simulink model "hdl_fft_sim"  (R2019a)
settings: Solver=VariableStepAuto  StartTime=0.0  StopTime=1024  RelTol=1e-3
undefined symbols (not defined in the file or in its folder): FFT, Wideband_FFT_slim
libraries: xbsIndex_r4 x22, casper_library_misc x1
settings Model: Creator=kocz  LastModifiedBy=kocz

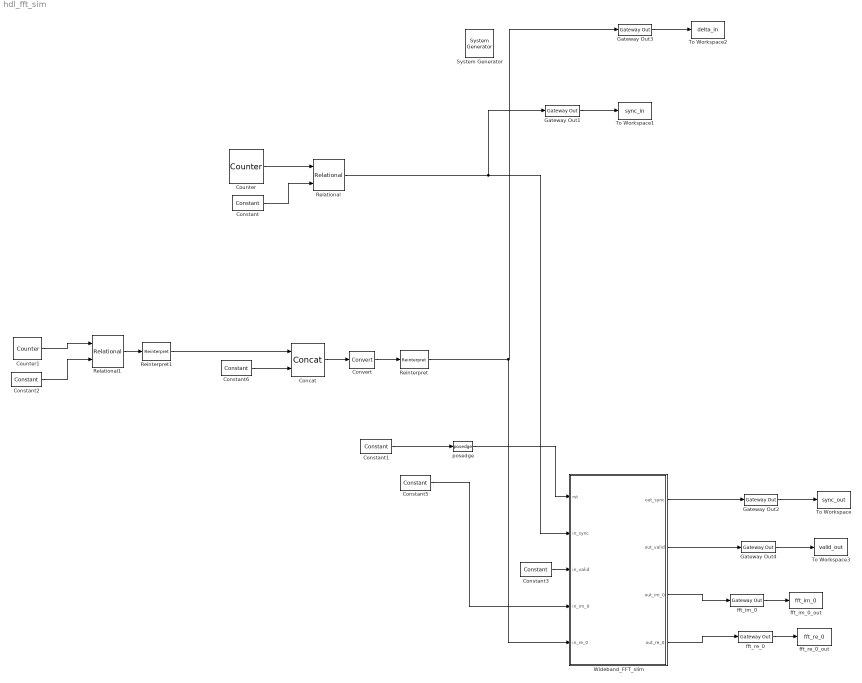
== system hdl_fft_sim ==
  " System Generator" : xbsIndex_r4/ System Generator  Tag=genX  xilinxfamily=kintex7  part=xc7k325t  speed=-3  package=fbg676  synthesis_tool=Vivado  clock_wrapper=Clock Enables  directory=./netlist  proj_type=Vivado  Synth_file=Vivado Synthesis Defaults  Impl_file=Vivado Implementation Defaults  testbench=off  simulink_period=1  sysclk_period=10  dcm_input_clock_period=10  incr_netlist=off  trim_vbits=Everywhere in SubSystem  dbl_ovrd=According to Block Masks  core_generation=According to Block Masks  run_coregen=off  deprecated_control=off  eval_field=0  block_type=sysgen
  Concat : xbsIndex_r4/Concat  num_inputs=2  dbl_ovrd=off  block_type=concat
  Constant : xbsIndex_r4/Constant  const=1  gui_display_data_type=Fixed-point  arith_type=Unsigned  n_bits=32  bin_pt=0  preci_type=Single  exp_width=8  frac_width=24  explicit_period=on  period=1  equ=P=C  opselect=C  inp2=PCIN>>17  opr=+  inp1=P  carry=CIN  dbl_ovrd=off  block_type=constant
  Constant1 : xbsIndex_r4/Constant  const=1  gui_display_data_type=Boolean  arith_type=Boolean  n_bits=16  bin_pt=14  preci_type=Single  exp_width=8  frac_width=24  explicit_period=on  period=1  equ=P=C  opselect=C  inp2=PCIN>>17  opr=+  inp1=P  carry=CIN  dbl_ovrd=off  block_type=constant
  Constant2 : xbsIndex_r4/Constant  const=1  gui_display_data_type=Fixed-point  arith_type=Unsigned  n_bits=32  bin_pt=0  preci_type=Single  exp_width=8  frac_width=24  explicit_period=on  period=1  equ=P=C  opselect=C  inp2=PCIN>>17  opr=+  inp1=P  carry=CIN  dbl_ovrd=off  block_type=constant
  Constant3 : xbsIndex_r4/Constant  const=1  gui_display_data_type=Boolean  arith_type=Boolean  n_bits=16  bin_pt=14  preci_type=Single  exp_width=8  frac_width=24  explicit_period=on  period=1  equ=P=C  opselect=C  inp2=PCIN>>17  opr=+  inp1=P  carry=CIN  dbl_ovrd=off  block_type=constant
  Constant5 : xbsIndex_r4/Constant  const=0  gui_display_data_type=Fixed-point  arith_type=Signed (2's comp)  n_bits=18  bin_pt=17  preci_type=Single  exp_width=8  frac_width=24  explicit_period=on  period=1  equ=P=C  opselect=C  inp2=PCIN>>17  opr=+  inp1=P  carry=CIN  dbl_ovrd=off  block_type=constant
  Constant6 : xbsIndex_r4/Constant  const=0  gui_display_data_type=Fixed-point  arith_type=Unsigned  n_bits=4  bin_pt=0  preci_type=Single  exp_width=8  frac_width=24  explicit_period=on  period=1  equ=P=C  opselect=C  inp2=PCIN>>17  opr=+  inp1=P  carry=CIN  dbl_ovrd=off  block_type=constant
  Convert : xbsIndex_r4/Convert  gui_display_data_type=Fixed-point  arith_type=Unsigned  n_bits=18  bin_pt=0  float_type=Single  exp_bits=8  fraction_bits=24  quantization=Truncate  overflow=Wrap  en=off  latency=2  pipeline=off  dbl_ovrd=off  block_type=convert
  Counter : xbsIndex_r4/Counter  cnt_type=Free Running  cnt_to=Inf  operation=Up  start_count=0  cnt_by_val=1  arith_type=Unsigned  n_bits=64  bin_pt=0  load_pin=off  rst=off  en=off  explicit_period=on  period=1  use_behavioral_HDL=off  implementation=Fabric  dbl_ovrd=off  block_type=counter
  Counter1 : xbsIndex_r4/Counter  cnt_type=Free Running  cnt_to=Inf  operation=Up  start_count=0  cnt_by_val=1  arith_type=Unsigned  n_bits=6  bin_pt=0  load_pin=off  rst=off  en=off  explicit_period=on  period=1  use_behavioral_HDL=off  implementation=Fabric  dbl_ovrd=off  block_type=counter
  Gateway Out{1..4} (4 alike) : xbsIndex_r4/Gateway Out  inherit_from_input=off  hdl_port=on  rows=1  columns=1  UseAsDAC=off  DACChannel='1'  interface=None  automatic_assignment=on  address_offset=hex2dec('00')  intf_name=''  intf_description=''  timing_constraint=None  locs_specified=off  LOCs={}  io_standard={}  block_type=gatewayout
  Reinterpret : xbsIndex_r4/Reinterpret  force_arith_type=on  arith_type="Signed  (2's comp)"  force_bin_pt=on  bin_pt=17  block_type=reinterpret
  Reinterpret1 : xbsIndex_r4/Reinterpret  force_arith_type=on  arith_type=Unsigned  force_bin_pt=on  bin_pt=0  block_type=reinterpret
  Relational : xbsIndex_r4/Relational  mode=a=b  op_type=Bool  en=off  latency=1  dbl_ovrd=off  block_type=relational
  Relational1 : xbsIndex_r4/Relational  mode=a=b  op_type=Bool  en=off  latency=0  dbl_ovrd=off  block_type=relational
  To Workspace : ToWorkspace  VariableName=sync_out  SampleTime=-1
      settings: Save2DSignal=2-D array (concatenate along first dimension)
  To Workspace1 : ToWorkspace  VariableName=sync_in  SampleTime=-1
      settings: Save2DSignal=2-D array (concatenate along first dimension)
  To Workspace2 : ToWorkspace  VariableName=delta_in  SampleTime=-1
      settings: Save2DSignal=2-D array (concatenate along first dimension)
  To Workspace3 : ToWorkspace  VariableName=valid_out  SampleTime=-1
      settings: Save2DSignal=2-D array (concatenate along first dimension)
  Wideband_FFT_slim : Subsystem  AncestorBlock=FFT/Wideband_FFT_slim  mask{use_separate=on, use_fft_shift=off, use_reorder=on, nof_chan=0, wb_factor=1, twiddle_offset=0, nof_points=1024, in_dat_w=8, out_dat_w=13, out_gain_w=0, stage_dat_w=16, guard_enable=off, guard_w=2, xtra_dat_sigs=off}
      mask prompts: use_separate "Separate complex in/out ports?"; use_fft_shift "Apply FFT shifting"; use_reorder "Reorder output"; nof_chan "Nof channels (time mux inputs)"; wb_factor "Wideband factor"; twiddle_offset "Twiddle offsets"; nof_points "Number of points"; in_dat_w "Input data width"; out_dat_w "Ouput data width"; out_gain_w "Output gain width"; stage_dat_w "Stage data width"; guard_enable "Guard enable"; guard_w "Guard bit width"; xtra_dat_sigs "Use extended data signals?"
      mask init:
      | Simulink.Block.eval([gcb, '/wb_fft_slim']);
      | 
      | wb_slim_subsys2bb_knit();
      | 
      | if strcmp(guard_enable,'on')
      |     guard_w = 2;
      | end
      mask Callback use_separate:
      | % Control parameter visiblity
      | 
      | % Get the value of the Enable Bias checkbox
      | % unchecked = 'off'
      | % checked = 'on'
      | enab = get_param(gcb,'use_separate');
      | 
      | % Set the 'MaskVisibilities' property for each parameters
      | if strcmp(enab,'on')
      |     set_param(gcb,'MaskEnables',{'on','off','off','on','on','on','on','on','on','on','on','on','on','on'});
      |     set_param(gcb,'use_reorder','on');
      |     set_param(gcb,'use_fft_shift','off');
      | else
      |     set_param(gcb,'MaskEnables',{'on','on','on','on','on','on','on','on','on','on','on','on','off','on'});
      | end
      | 
      | % Note that the value of the bias is not handled here.
      | % See the Initialization tab
      mask Callback use_fft_shift:
      | % Control parameter visiblity
      | 
      | % Get the value of the Enable Bias checkbox
      | % unchecked = 'off'
      | % checked = 'on'
      | enab = get_param(gcb,'use_fft_shift');
      | 
      | % Set the 'MaskVisibilities' property for each parameters
      | if strcmp(enab,'on')
      |     set_param(gcb,'MaskEnables',{'on','on','off','on','on','on','on','on','on','on','on','on','off','on'});
      |     set_param(gcb,'use_reorder','on');
      | else
      |     set_param(gcb,'MaskEnables',{'on','on','on','on','on','on','on','on','on','on','on','on','off','on'});
      | end
      | 
      | % Note that the value of the bias is not handled here.
      | % See the Initialization tab
      mask Callback guard_enable:
      | % Control parameter visiblity
      | 
      | % Get the value of the Enable Bias checkbox
      | % unchecked = 'off'
      | % checked = 'on'
      | enab = get_param(gcb,'guard_enable');
      | 
      | % Set the 'MaskVisibilities' property for each parameters
      | if strcmp(enab,'on')
      |     set_param(gcb,'MaskVisibilities',{'on','on','on','on','on','on','on','on','on','on','on','on','on','on'});
      | else
      |     set_param(gcb,'MaskVisibilities',{'on','on','on','on','on','on','on','on','on','on','on','on','off','on'});
      | end
      | 
      | % Note that the value of the bias is not handled here.
      | % See the Initialization tab
  fft_im_0 : xbsIndex_r4/Gateway Out  inherit_from_input=off  hdl_port=on  rows=1  columns=1  UseAsDAC=off  DACChannel='1'  interface=None  automatic_assignment=on  address_offset=hex2dec('00')  intf_name=''  intf_description=''  timing_constraint=None  locs_specified=off  LOCs={}  io_standard={}  block_type=gatewayout
  fft_im_0_out : ToWorkspace  VariableName=fft_im_0  SampleTime=-1
      settings: Save2DSignal=2-D array (concatenate along first dimension)
  fft_re_0 : xbsIndex_r4/Gateway Out  inherit_from_input=off  hdl_port=on  rows=1  columns=1  UseAsDAC=off  DACChannel='1'  interface=None  automatic_assignment=on  address_offset=hex2dec('00')  intf_name=''  intf_description=''  timing_constraint=None  locs_specified=off  LOCs={}  io_standard={}  block_type=gatewayout
  fft_re_0_out : ToWorkspace  VariableName=fft_re_0  SampleTime=-1
      settings: Save2DSignal=2-D array (concatenate along first dimension)
  posedge : casper_library_misc/posedge  Tag=Rising Edge Detector
      settings: SourceProductName=CASPER DSP Blockset
  wires:
  Wideband_FFT_slim/1(out_sync) -> Gateway Out2/1
  Wideband_FFT_slim/4(out_re_0) -> fft_re_0/1
  Wideband_FFT_slim/3(out_im_0) -> fft_im_0/1
  fft_re_0/1 -> fft_re_0_out/1
  fft_im_0/1 -> fft_im_0_out/1
  Constant/1 -> Relational/2
  Counter/1 -> Relational/1
  Relational/1 -> Wideband_FFT_slim/2(in_sync), Gateway Out1/1
  Counter1/1 -> Relational1/1
  Constant2/1 -> Relational1/2
  Convert/1 -> Reinterpret/1
  Gateway Out2/1 -> To Workspace/1
  Concat/1 -> Convert/1
  Relational1/1 -> Reinterpret1/1
  Reinterpret1/1 -> Concat/1
  Constant6/1 -> Concat/2
  Gateway Out1/1 -> To Workspace1/1
  Gateway Out3/1 -> To Workspace2/1
  Reinterpret/1 -> Wideband_FFT_slim/5(in_re_0), Gateway Out3/1
  Constant5/1 -> Wideband_FFT_slim/4(in_im_0)
  Constant1/1 -> posedge/1
  posedge/1 -> Wideband_FFT_slim/1(rst)
  Constant3/1 -> Wideband_FFT_slim/3(in_valid)
  Gateway Out4/1 -> To Workspace3/1
  Wideband_FFT_slim/2(out_valid) -> Gateway Out4/1

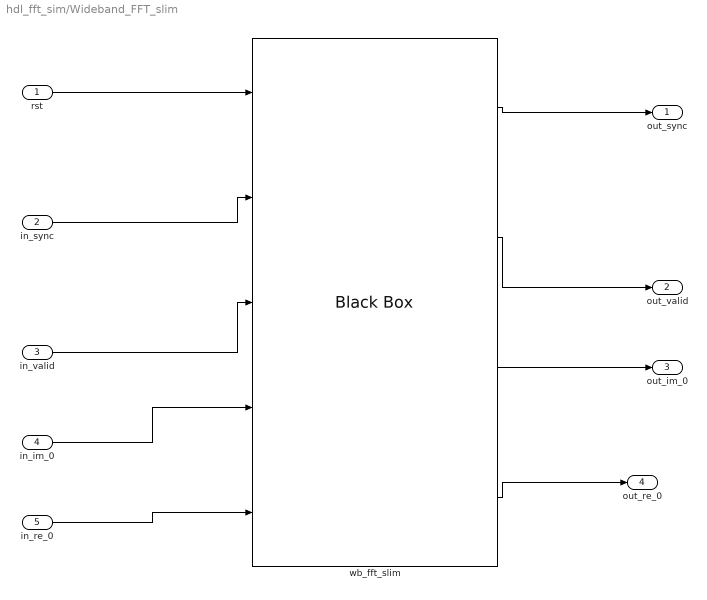
== system hdl_fft_sim/Wideband_FFT_slim ==
  rst : Inport
  in_sync : Inport  Port=2
  in_valid : Inport  Port=3
  in_im_0 : Inport  Port=4
  in_re_0 : Inport  Port=5
  wb_fft_slim : xbsIndex_r4/Black Box  init_code=wideband_fft_slim_top_config  sim_method=ISE Simulator  verbose=off  block_type=blackbox2
  out_sync : Outport
  out_valid : Outport  Port=2
  out_im_0 : Outport  Port=3
  out_re_0 : Outport  Port=4
  wires:
  wb_fft_slim/4 -> out_re_0/1
  wb_fft_slim/3 -> out_im_0/1
  in_re_0/1 -> wb_fft_slim/5
  in_im_0/1 -> wb_fft_slim/4
  wb_fft_slim/2 -> out_valid/1
  in_valid/1 -> wb_fft_slim/3
  wb_fft_slim/1 -> out_sync/1
  in_sync/1 -> wb_fft_slim/2
  rst/1 -> wb_fft_slim/1
